simulink model "NN_PID"  (R2015a)
settings: Solver=ode45  StartTime=0.0  StopTime=40  FixedStep=0.001  RelTol=1e-3
libraries: neural x141, simulink x18, commnoisgen2 x5
(part 4 of 5)

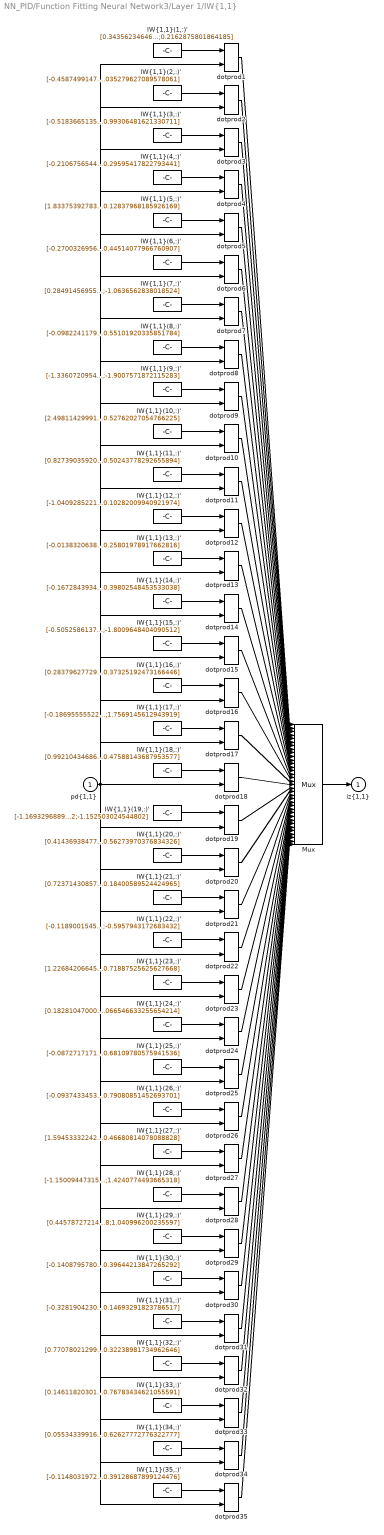
== system NN_PID/Function Fitting Neural Network3/Layer 1/IW{1,1} ==
  "pd{1,1}" : Inport  PortDimensions=20
      mask Display: e = 0.06;c1 = [120 230 180]/255;c2 = ([120 230 180]+0)/(256+128);c3 = ([120 230 180]+128)/(256+128);patch([0 1 1 0],[0 0 1 1],c1);patch([0 1 1 1-e 1-e 0+e],[0 0 1 1-e 0+e 0+e],c2);patch([0 0 1 1-e 0+e 0+e],[0 1 1 1-e 1-e 0+e],c3);plot([0 1 1 0 0],[0 0 1 1 0]);
  "IW{1,1}(1,:)'" : Constant  Value=[0.34356234646692452;0.21075488404779572;-0.32918291490554014;-0.32160977511543937;0.053207015633117721;0.43412666767247687;0.41202936590274203;0.39636100711472483;0.37639200502517606;-0.20160585970954958;0.2178319201514245;-0.15520948631781495;0.41615739491474962;-0.51184357545666392;0.38003175420582036;-0.50663702446248604;-0.33099837520790598;0.23966865807280641;0.30544580093767087;0.2162875801864185]
      mask Display: e = 0.06;c1 = [120 150 230]/255;c2 = ([120 150 230]+0)/383;c3 = ([120 150 230]+128)/383;patch([0 1 1 0],[0 0 1 1],c1);patch([0 1 1 1-e 1-e 0+e],[0 0 1 1-e 0+e 0+e],c2);patch([0 0 1 1-e 0+e 0+e],[0 1 1 1-e 1-e 0+e],c3);plot([0 1 1 0 0],[0 0 1 1 0]);disp('Weights');
  "IW{1,1}(10,:)'" : Constant  Value=[2.4981142999171224;-0.480167607602763;-0.23996584207603056;-0.53354314175989903;0.93267988161096238;-1.7895899467096461;-0.4490755724887166;-0.72970836466593303;1.6629857299245596;-1.9396925626168768;-0.017505824223907049;-0.031299172514314889;1.1546750149237817;-1.6466507506149892;0.20695638652045692;-0.69381111882218005;1.1318302015599122;-0.29293625128375828;0.58881496104867304;0.52762027054766225]
      mask Display: e = 0.06;c1 = [120 150 230]/255;c2 = ([120 150 230]+0)/383;c3 = ([120 150 230]+128)/383;patch([0 1 1 0],[0 0 1 1],c1);patch([0 1 1 1-e 1-e 0+e],[0 0 1 1-e 0+e 0+e],c2);patch([0 0 1 1-e 0+e 0+e],[0 1 1 1-e 1-e 0+e],c3);plot([0 1 1 0 0],[0 0 1 1 0]);disp('Weights');
  "IW{1,1}(11,:)'" : Constant  Value=[0.82739035920591841;0.077847341769124334;0.16416721969600542;1.3190138770003537;0.51689708649492772;0.13414226906759166;0.67634139729661547;0.29270384872245042;0.53460787889922456;0.01047726123783488;0.95499156644453731;0.15165043809919779;-0.46476741210461053;0.65252713334295698;-0.23470786792487017;0.17785522832461254;0.15426082557036538;0.51671816474315135;0.57531946627955011;-0.50243778292655894]
      mask Display: e = 0.06;c1 = [120 150 230]/255;c2 = ([120 150 230]+0)/383;c3 = ([120 150 230]+128)/383;patch([0 1 1 0],[0 0 1 1],c1);patch([0 1 1 1-e 1-e 0+e],[0 0 1 1-e 0+e 0+e],c2);patch([0 0 1 1-e 0+e 0+e],[0 1 1 1-e 1-e 0+e],c3);plot([0 1 1 0 0],[0 0 1 1 0]);disp('Weights');
  "IW{1,1}(12,:)'" : Constant  Value=[-1.0409285221258437;1.1150835262775509;-0.13810878388359787;-0.48646754358867977;-0.93383972503414348;1.572249478067455;0.25639929226933394;-0.38439956059154529;-0.70061918501654008;1.1204888375798943;0.13613187983183514;-0.58583571435844506;-1.4949035051599902;1.1826688812367208;-0.16589964378960401;-0.27085123700682673;-1.5697903319513054;0.53372313151016015;-0.20298933792670701;-0.10282009940921974]
      mask Display: e = 0.06;c1 = [120 150 230]/255;c2 = ([120 150 230]+0)/383;c3 = ([120 150 230]+128)/383;patch([0 1 1 0],[0 0 1 1],c1);patch([0 1 1 1-e 1-e 0+e],[0 0 1 1-e 0+e 0+e],c2);patch([0 0 1 1-e 0+e 0+e],[0 1 1 1-e 1-e 0+e],c3);plot([0 1 1 0 0],[0 0 1 1 0]);disp('Weights');
  "IW{1,1}(13,:)'" : Constant  Value=[-0.013832063818641063;-0.93403249848454817;-0.18601282121761561;-0.02167639873884359;0.51876133590062801;0.62596273151480519;-0.33256901492513785;0.20690823337916611;0.56369902073090317;-0.2353309824929046;0.42254575942954581;0.056199503759795696;-0.48952800638643007;-0.33465615368609403;0.490489950428382;0.50817783817270235;-0.33952374105593836;0.60950502388303041;-0.48972816769454419;-0.25801978917662816]
      mask Display: e = 0.06;c1 = [120 150 230]/255;c2 = ([120 150 230]+0)/383;c3 = ([120 150 230]+128)/383;patch([0 1 1 0],[0 0 1 1],c1);patch([0 1 1 1-e 1-e 0+e],[0 0 1 1-e 0+e 0+e],c2);patch([0 0 1 1-e 0+e 0+e],[0 1 1 1-e 1-e 0+e],c3);plot([0 1 1 0 0],[0 0 1 1 0]);disp('Weights');
  "IW{1,1}(14,:)'" : Constant  Value=[-0.16728439348193508;0.11201921876606614;-0.84717081620446133;0.033643437188791349;0.073870720164509712;0.23557579873900267;-0.47069890579339591;-0.048283879330601416;0.62682672795060768;0.3856976010503208;-1.0937018076565657;-0.24568147821005917;0.36176114292675432;0.0030879549749601026;-0.19797420086140236;0.62609705792546555;0.47665621841435707;-0.17765647171953722;0.33716085953108443;0.39802548453533038]
      mask Display: e = 0.06;c1 = [120 150 230]/255;c2 = ([120 150 230]+0)/383;c3 = ([120 150 230]+128)/383;patch([0 1 1 0],[0 0 1 1],c1);patch([0 1 1 1-e 1-e 0+e],[0 0 1 1-e 0+e 0+e],c2);patch([0 0 1 1-e 0+e 0+e],[0 1 1 1-e 1-e 0+e],c3);plot([0 1 1 0 0],[0 0 1 1 0]);disp('Weights');
  "IW{1,1}(15,:)'" : Constant  Value=[-0.50525861373297221;-0.50234172039067404;-1.0214503230073055;-0.73512099097471728;-0.88924848549223867;0.5719133518109677;-1.0086133763648022;-0.1232185415699124;-1.2092925802018386;0.097016377172541302;-0.31259485998115577;-0.38420476108191332;-0.96541704936768968;-0.79100586037197529;-0.44049745783924749;-0.23874302342060633;-0.53384968992013559;-1.0556645069035904;-1.5346677460116795;-1.8009648404090512]
      mask Display: e = 0.06;c1 = [120 150 230]/255;c2 = ([120 150 230]+0)/383;c3 = ([120 150 230]+128)/383;patch([0 1 1 0],[0 0 1 1],c1);patch([0 1 1 1-e 1-e 0+e],[0 0 1 1-e 0+e 0+e],c2);patch([0 0 1 1-e 0+e 0+e],[0 1 1 1-e 1-e 0+e],c3);plot([0 1 1 0 0],[0 0 1 1 0]);disp('Weights');
  "IW{1,1}(16,:)'" : Constant  Value=[0.28379627729071083;0.017475468939408212;0.78742097530841404;0.3402729448293319;-0.03791020600260353;0.24793319509467407;-0.14680536026554428;-0.13246445638569912;0.87176237899940057;-0.38188832490596736;0.10689208200390865;0.3257288375296703;0.076245952530720834;-0.7072342525186468;-0.54396222693874152;-0.35344510808923141;-0.559401986937623;0.39483752858509835;0.027810353114642975;0.37325192473166446]
      mask Display: e = 0.06;c1 = [120 150 230]/255;c2 = ([120 150 230]+0)/383;c3 = ([120 150 230]+128)/383;patch([0 1 1 0],[0 0 1 1],c1);patch([0 1 1 1-e 1-e 0+e],[0 0 1 1-e 0+e 0+e],c2);patch([0 0 1 1-e 0+e 0+e],[0 1 1 1-e 1-e 0+e],c3);plot([0 1 1 0 0],[0 0 1 1 0]);disp('Weights');
  "IW{1,1}(17,:)'" : Constant  Value=[-0.18695555522388208;1.1457766997082237;1.8932469743660993;1.2091852348847023;2.1793357647278508;1.5715364071793236;0.93546861520022606;1.1462136972388943;1.5547425674166264;2.1035568853621531;0.31032076523265922;-0.64150014048513371;0.98292572222818919;3.4684809472989642;1.449667710887623;2.0822190456442886;0.52834723860767396;3.448326587365893;0.66275802173830167;1.7569145612943919]
      mask Display: e = 0.06;c1 = [120 150 230]/255;c2 = ([120 150 230]+0)/383;c3 = ([120 150 230]+128)/383;patch([0 1 1 0],[0 0 1 1],c1);patch([0 1 1 1-e 1-e 0+e],[0 0 1 1-e 0+e 0+e],c2);patch([0 0 1 1-e 0+e 0+e],[0 1 1 1-e 1-e 0+e],c3);plot([0 1 1 0 0],[0 0 1 1 0]);disp('Weights');
  "IW{1,1}(18,:)'" : Constant  Value=[0.99210434686555449;-0.19182862219447805;0.83496313248633269;0.82543212806801092;-0.48831989615704796;0.17785622865467884;-0.44052762940670648;-0.93383095450336107;-1.1799218338811521;0.14631114551825533;-0.98018487699314072;-0.73495232655399023;-1.1740161013384385;0.40195376720796966;-0.68300841779666577;-0.94937235867190894;-0.72509839269384035;-0.36381020107243528;-0.56716335450951727;-0.47588143687953577]
      mask Display: e = 0.06;c1 = [120 150 230]/255;c2 = ([120 150 230]+0)/383;c3 = ([120 150 230]+128)/383;patch([0 1 1 0],[0 0 1 1],c1);patch([0 1 1 1-e 1-e 0+e],[0 0 1 1-e 0+e 0+e],c2);patch([0 0 1 1-e 0+e 0+e],[0 1 1 1-e 1-e 0+e],c3);plot([0 1 1 0 0],[0 0 1 1 0]);disp('Weights');
  "IW{1,1}(19,:)'" : Constant  Value=[-1.1693296889016684;-0.74637919668481101;-0.080745252440748996;-0.73555456972101541;-1.3624453036065594;-0.6245328994526842;-0.27615182737914001;-0.32223288713346271;-1.1053147331161475;-1.5638418877440929;0.040201830826049452;-0.69568617475109829;-1.4771542884699433;-1.384562078451685;-0.72957057859092778;-1.1255661172123617;-2.0769672387096767;-1.5456121624405867;-1.7004814221851852;-1.152503024544802]
      mask Display: e = 0.06;c1 = [120 150 230]/255;c2 = ([120 150 230]+0)/383;c3 = ([120 150 230]+128)/383;patch([0 1 1 0],[0 0 1 1],c1);patch([0 1 1 1-e 1-e 0+e],[0 0 1 1-e 0+e 0+e],c2);patch([0 0 1 1-e 0+e 0+e],[0 1 1 1-e 1-e 0+e],c3);plot([0 1 1 0 0],[0 0 1 1 0]);disp('Weights');
  "IW{1,1}(2,:)'" : Constant  Value=[-0.45874991478413735;-0.48613190251108701;-0.58937576807537073;-0.23422038712857843;-0.38105537807544038;0.15036490759582355;-0.00046876757349376651;0.4827296218033143;0.054361047774846384;0.023237702645422229;0.31821604735154824;-0.24689697381512252;0.53417251129328136;-0.46757684959937867;0.42729361373870245;-0.57415192726693309;-0.46080164770445725;0.43650630863441764;-0.0049774707672980579;0.035279627089578061]
      mask Display: e = 0.06;c1 = [120 150 230]/255;c2 = ([120 150 230]+0)/383;c3 = ([120 150 230]+128)/383;patch([0 1 1 0],[0 0 1 1],c1);patch([0 1 1 1-e 1-e 0+e],[0 0 1 1-e 0+e 0+e],c2);patch([0 0 1 1-e 0+e 0+e],[0 1 1 1-e 1-e 0+e],c3);plot([0 1 1 0 0],[0 0 1 1 0]);disp('Weights');
  "IW{1,1}(20,:)'" : Constant  Value=[0.41436938477688684;0.19335022646292935;0.014772848406684008;-0.13512928805120403;-0.063179445899241182;-0.42957513089188293;0.19337496274880683;-0.1363777958223984;0.37708859412077506;-0.025121212643982049;-0.51392570544386584;0.22904057847712325;-0.61118914251844358;0.034674346520921023;-0.41877101993291993;0.31715794586772383;0.56103736438551832;-0.01670095701532218;-0.40421432346150343;-0.56273970376834326]
      mask Display: e = 0.06;c1 = [120 150 230]/255;c2 = ([120 150 230]+0)/383;c3 = ([120 150 230]+128)/383;patch([0 1 1 0],[0 0 1 1],c1);patch([0 1 1 1-e 1-e 0+e],[0 0 1 1-e 0+e 0+e],c2);patch([0 0 1 1-e 0+e 0+e],[0 1 1 1-e 1-e 0+e],c3);plot([0 1 1 0 0],[0 0 1 1 0]);disp('Weights');
  "IW{1,1}(21,:)'" : Constant  Value=[0.72371430857203933;-3.593614507511715;-4.5871449552524277;-4.2122412121628168;0.6399350416139965;-1.818477312716956;-1.2906611084941901;-1.2875356240111187;1.123659568248192;4.3159262343879039;4.159305627556579;4.3607458437542546;0.070723338557161675;1.883176982219871;1.3223080957068787;0.86829251394765461;0.061714721775943823;0.82510572719976227;0.024549786069301308;0.18400589524424965]
      mask Display: e = 0.06;c1 = [120 150 230]/255;c2 = ([120 150 230]+0)/383;c3 = ([120 150 230]+128)/383;patch([0 1 1 0],[0 0 1 1],c1);patch([0 1 1 1-e 1-e 0+e],[0 0 1 1-e 0+e 0+e],c2);patch([0 0 1 1-e 0+e 0+e],[0 1 1 1-e 1-e 0+e],c3);plot([0 1 1 0 0],[0 0 1 1 0]);disp('Weights');
  "IW{1,1}(22,:)'" : Constant  Value=[-0.11890015452014127;-0.687701181255719;0.94376206362901938;0.23081451882508561;0.043195706054232758;0.09612049266731798;-1.1065870947943734;-0.34467190237267864;0.37138161986991153;-0.035530615058210979;-0.12065594561795193;-0.22772992194836639;0.052864999454783623;0.24879892992991279;-0.10384812085318716;-0.87109233921532081;-0.27939576841829955;0.20517011822505235;-0.16563869623528174;-0.5957943172683432]
      mask Display: e = 0.06;c1 = [120 150 230]/255;c2 = ([120 150 230]+0)/383;c3 = ([120 150 230]+128)/383;patch([0 1 1 0],[0 0 1 1],c1);patch([0 1 1 1-e 1-e 0+e],[0 0 1 1-e 0+e 0+e],c2);patch([0 0 1 1-e 0+e 0+e],[0 1 1 1-e 1-e 0+e],c3);plot([0 1 1 0 0],[0 0 1 1 0]);disp('Weights');
  "IW{1,1}(23,:)'" : Constant  Value=[1.2268420664527899;-4.7473520608111759;-4.5111987662169808;-4.1301102543078345;0.95314682285552443;-1.5369554180305878;-1.2194928954807696;-1.48885521534928;0.69535722255434684;1.1269711738240547;0.42081703079226829;-0.11006423540082071;-0.23153805097746277;3.4870735970031581;4.5861277082200518;4.686153128178999;0.23984369369556707;1.6628058364914811;0.92075306018939429;0.71887525625627668]
      mask Display: e = 0.06;c1 = [120 150 230]/255;c2 = ([120 150 230]+0)/383;c3 = ([120 150 230]+128)/383;patch([0 1 1 0],[0 0 1 1],c1);patch([0 1 1 1-e 1-e 0+e],[0 0 1 1-e 0+e 0+e],c2);patch([0 0 1 1-e 0+e 0+e],[0 1 1 1-e 1-e 0+e],c3);plot([0 1 1 0 0],[0 0 1 1 0]);disp('Weights');
  "IW{1,1}(24,:)'" : Constant  Value=[0.1828104700025977;0.31176410854197356;0.40962405803784929;-0.35642553788699693;0.057716522600453353;-0.14874504578074377;0.21254620417334505;0.46042974283685917;0.35404341798226119;0.54172712136154977;-0.58235172545159641;0.64388708858811594;-0.085376147584756507;-0.13314351100017599;-0.82733218028564015;-0.31607893422153477;0.13665134877093729;0.50278509641500502;-0.49743935447695131;0.066546633255654214]
      mask Display: e = 0.06;c1 = [120 150 230]/255;c2 = ([120 150 230]+0)/383;c3 = ([120 150 230]+128)/383;patch([0 1 1 0],[0 0 1 1],c1);patch([0 1 1 1-e 1-e 0+e],[0 0 1 1-e 0+e 0+e],c2);patch([0 0 1 1-e 0+e 0+e],[0 1 1 1-e 1-e 0+e],c3);plot([0 1 1 0 0],[0 0 1 1 0]);disp('Weights');
  "IW{1,1}(25,:)'" : Constant  Value=[-0.087271717146533007;0.11846226575201743;-0.88849593889350431;0.01343112444477061;0.23506583523325256;-0.55234171611056559;-0.47407407395654277;-0.89033223489029933;0.32638481951364251;0.085735419140751196;0.19454675867100721;0.16352631936097936;0.24207477015981532;0.40002761318930891;-0.43910346364545572;-0.084180568243685763;0.20417455686475997;0.29556820825651187;-0.9555995930734853;-0.68109780575941536]
      mask Display: e = 0.06;c1 = [120 150 230]/255;c2 = ([120 150 230]+0)/383;c3 = ([120 150 230]+128)/383;patch([0 1 1 0],[0 0 1 1],c1);patch([0 1 1 1-e 1-e 0+e],[0 0 1 1-e 0+e 0+e],c2);patch([0 0 1 1-e 0+e 0+e],[0 1 1 1-e 1-e 0+e],c3);plot([0 1 1 0 0],[0 0 1 1 0]);disp('Weights');
  "IW{1,1}(26,:)'" : Constant  Value=[-0.09374334534187008;1.3244361403553937;-0.63214199309847263;-0.8046250420468043;-0.12004482527427369;1.4122826750950541;-0.46195733135223244;-0.33569199429964125;0.6723514281939984;0.7757678158200717;-0.12247575393999316;-0.67933129844318407;0.49379968478505742;1.1284426114223642;-0.12646136822926446;-0.96154617316407409;0.4222472421730753;1.7752297376962451;-0.2198145398921153;0.79080851452693701]
      mask Display: e = 0.06;c1 = [120 150 230]/255;c2 = ([120 150 230]+0)/383;c3 = ([120 150 230]+128)/383;patch([0 1 1 0],[0 0 1 1],c1);patch([0 1 1 1-e 1-e 0+e],[0 0 1 1-e 0+e 0+e],c2);patch([0 0 1 1-e 0+e 0+e],[0 1 1 1-e 1-e 0+e],c3);plot([0 1 1 0 0],[0 0 1 1 0]);disp('Weights');
  "IW{1,1}(27,:)'" : Constant  Value=[1.5945333224281737;0.55750703331793905;0.22834970803469309;-0.55407924594364444;1.0159402558435906;0.13475888457100102;-0.94932585473437592;-0.57833908101215381;-0.21137194482521771;0.50264147781836055;-0.71057721429377341;-0.53496766081529434;0.92991557220437915;0.035881786802091149;-0.12810043583382549;0.47563250604500451;0.70661794378473586;0.15093136252852452;-0.26867178952295967;0.46680814078088828]
      mask Display: e = 0.06;c1 = [120 150 230]/255;c2 = ([120 150 230]+0)/383;c3 = ([120 150 230]+128)/383;patch([0 1 1 0],[0 0 1 1],c1);patch([0 1 1 1-e 1-e 0+e],[0 0 1 1-e 0+e 0+e],c2);patch([0 0 1 1-e 0+e 0+e],[0 1 1 1-e 1-e 0+e],c3);plot([0 1 1 0 0],[0 0 1 1 0]);disp('Weights');
  "IW{1,1}(28,:)'" : Constant  Value=[-1.1500944731533365;-0.43882767108252868;-0.51887067559486078;-0.21705590803186423;0.64998926612131047;0.074724502831834599;0.51817566210952459;0.15966122964102833;-0.5305213838452506;-0.64232198762760617;0.019688137381493213;0.7101963909482143;0.50278728648409843;-0.50395246145283856;-0.0384367465017523;0.7006560242347899;0.74282118842488443;-0.3092943056200102;1.132192267381624;1.4240774493665318]
      mask Display: e = 0.06;c1 = [120 150 230]/255;c2 = ([120 150 230]+0)/383;c3 = ([120 150 230]+128)/383;patch([0 1 1 0],[0 0 1 1],c1);patch([0 1 1 1-e 1-e 0+e],[0 0 1 1-e 0+e 0+e],c2);patch([0 0 1 1-e 0+e 0+e],[0 1 1 1-e 1-e 0+e],c3);plot([0 1 1 0 0],[0 0 1 1 0]);disp('Weights');
  "IW{1,1}(29,:)'" : Constant  Value=[0.4457872721469528;0.58517860925478815;1.5198138112088939;1.3388659684533255;1.0846180372345164;1.1710924821688653;0.20580558202619828;0.68665967354208979;0.78124105378263409;1.4629040401659914;0.18650798192964127;-0.28169842008850166;2.2921228518259875;1.336080981220338;0.63273574394653065;1.520874114106693;1.7567076375137654;1.9649644914451438;1.5521312330859938;1.040996200235597]
      mask Display: e = 0.06;c1 = [120 150 230]/255;c2 = ([120 150 230]+0)/383;c3 = ([120 150 230]+128)/383;patch([0 1 1 0],[0 0 1 1],c1);patch([0 1 1 1-e 1-e 0+e],[0 0 1 1-e 0+e 0+e],c2);patch([0 0 1 1-e 0+e 0+e],[0 1 1 1-e 1-e 0+e],c3);plot([0 1 1 0 0],[0 0 1 1 0]);disp('Weights');
  "IW{1,1}(3,:)'" : Constant  Value=[-0.51836651359350794;0.16692147273010965;0.031973839099968066;-0.26285055514279515;0.28220541671325394;-0.31185493096221517;0.02025865629207203;0.32669005765432318;0.0030836598159332731;-0.30832253903406404;-0.060331423326532442;0.73993666609635833;-0.56256953169833701;-0.70698345300566645;0.12808614394253007;0.14122723182564098;-0.48637830190550663;-0.62391538238897659;0.53003124334445673;0.99306481621330711]
      mask Display: e = 0.06;c1 = [120 150 230]/255;c2 = ([120 150 230]+0)/383;c3 = ([120 150 230]+128)/383;patch([0 1 1 0],[0 0 1 1],c1);patch([0 1 1 1-e 1-e 0+e],[0 0 1 1-e 0+e 0+e],c2);patch([0 0 1 1-e 0+e 0+e],[0 1 1 1-e 1-e 0+e],c3);plot([0 1 1 0 0],[0 0 1 1 0]);disp('Weights');
  "IW{1,1}(30,:)'" : Constant  Value=[-0.14087957801899462;0.35478617648225291;0.21149403522513699;0.41056377044908776;-0.22087054921988736;0.33497419776735021;-0.47436486406119416;-0.21221549723051042;-0.13432546537312118;0.13701637376577269;0.57805578395562429;-0.45610077329690285;0.34376937107205774;0.14500638232797852;0.44278206811243981;0.48664218987103935;0.072347278241116419;-0.24825374179427259;0.35229824512171154;-0.39644213847265292]
      mask Display: e = 0.06;c1 = [120 150 230]/255;c2 = ([120 150 230]+0)/383;c3 = ([120 150 230]+128)/383;patch([0 1 1 0],[0 0 1 1],c1);patch([0 1 1 1-e 1-e 0+e],[0 0 1 1-e 0+e 0+e],c2);patch([0 0 1 1-e 0+e 0+e],[0 1 1 1-e 1-e 0+e],c3);plot([0 1 1 0 0],[0 0 1 1 0]);disp('Weights');
  "IW{1,1}(31,:)'" : Constant  Value=[-0.32819042308196561;-0.10257381139188286;-0.37073977541966974;0.22423958924412016;-0.30795253328795763;-0.2071706128605553;-0.29040709456208469;0.082390531186220389;0.024067580871069288;0.10355229251895358;-0.13442658112358469;-0.36892314629287865;0.0045907106848744519;0.14032411420945257;-0.63942121124786999;0.15469183047235713;0.22767133858986385;-0.84477672859441388;-0.52904942613742845;0.14693291823786517]
      mask Display: e = 0.06;c1 = [120 150 230]/255;c2 = ([120 150 230]+0)/383;c3 = ([120 150 230]+128)/383;patch([0 1 1 0],[0 0 1 1],c1);patch([0 1 1 1-e 1-e 0+e],[0 0 1 1-e 0+e 0+e],c2);patch([0 0 1 1-e 0+e 0+e],[0 1 1 1-e 1-e 0+e],c3);plot([0 1 1 0 0],[0 0 1 1 0]);disp('Weights');
  "IW{1,1}(32,:)'" : Constant  Value=[0.77078021299402288;0.48081029505425493;0.21396388817095;0.12098863491066988;-0.055146482277161582;-0.39346723996023797;-0.53265112102000001;0.63390013940259193;-0.070239993932744618;0.39147026707548149;-0.12335078085922772;0.030639159154381899;-0.11383942996015066;-0.11289035557254473;-0.080150625413985321;-0.05715888336882638;0.3149151289412182;0.77859308616016143;0.085079172258503657;-0.32238981734962646]
      mask Display: e = 0.06;c1 = [120 150 230]/255;c2 = ([120 150 230]+0)/383;c3 = ([120 150 230]+128)/383;patch([0 1 1 0],[0 0 1 1],c1);patch([0 1 1 1-e 1-e 0+e],[0 0 1 1-e 0+e 0+e],c2);patch([0 0 1 1-e 0+e 0+e],[0 1 1 1-e 1-e 0+e],c3);plot([0 1 1 0 0],[0 0 1 1 0]);disp('Weights');
  "IW{1,1}(33,:)'" : Constant  Value=[0.14611820301917341;0.64966054747678437;-0.42060935671336647;-0.4822177238213004;-0.3443061873458565;0.67872546150737856;-1.2961091025588496;-0.85405600467188114;0.4144326914735576;-0.49244428450591682;-0.61602028085161153;-1.404689011803915;0.036698519057189002;-0.1393109837722625;0.23336169055112679;-0.32375828832886511;-0.32272519052731796;-0.34853452171972116;-0.013253958950352413;-0.76783434621055591]
      mask Display: e = 0.06;c1 = [120 150 230]/255;c2 = ([120 150 230]+0)/383;c3 = ([120 150 230]+128)/383;patch([0 1 1 0],[0 0 1 1],c1);patch([0 1 1 1-e 1-e 0+e],[0 0 1 1-e 0+e 0+e],c2);patch([0 0 1 1-e 0+e 0+e],[0 1 1 1-e 1-e 0+e],c3);plot([0 1 1 0 0],[0 0 1 1 0]);disp('Weights');
  "IW{1,1}(34,:)'" : Constant  Value=[0.055343399162782109;0.24967641914961913;0.22849492051757608;-0.2583701706610419;0.30234756432963239;-0.48373279085941684;-0.66349211767724392;-0.11638829875459623;0.1204720283996237;0.11020238984962738;0.48558152277647532;-0.39019701281895142;0.13510202742216729;0.23181593998038813;0.34658478847348279;0.53070352063144199;-0.40685898175808061;-0.44530896115461038;0.16484066077329629;-0.62627772776322777]
      mask Display: e = 0.06;c1 = [120 150 230]/255;c2 = ([120 150 230]+0)/383;c3 = ([120 150 230]+128)/383;patch([0 1 1 0],[0 0 1 1],c1);patch([0 1 1 1-e 1-e 0+e],[0 0 1 1-e 0+e 0+e],c2);patch([0 0 1 1-e 0+e 0+e],[0 1 1 1-e 1-e 0+e],c3);plot([0 1 1 0 0],[0 0 1 1 0]);disp('Weights');
  "IW{1,1}(35,:)'" : Constant  Value=[-0.11480319726314336;-0.5806357619062531;0.07252454074519965;-0.33034408197078352;-0.3570814673011331;-0.2053356453621932;0.055913137533546028;-0.15679935021763422;0.2825223410388083;0.35167845327504432;-0.16986653971270321;0.40801261453603693;-0.49009057489775432;0.38190469377654135;0.13229706695680551;0.45226062586800231;-0.41911899832237653;-0.25532488945121812;-0.49875611392974706;0.39128687899124476]
      mask Display: e = 0.06;c1 = [120 150 230]/255;c2 = ([120 150 230]+0)/383;c3 = ([120 150 230]+128)/383;patch([0 1 1 0],[0 0 1 1],c1);patch([0 1 1 1-e 1-e 0+e],[0 0 1 1-e 0+e 0+e],c2);patch([0 0 1 1-e 0+e 0+e],[0 1 1 1-e 1-e 0+e],c3);plot([0 1 1 0 0],[0 0 1 1 0]);disp('Weights');
  "IW{1,1}(4,:)'" : Constant  Value=[-0.21067565440528216;-0.16639612349532221;-0.89778075327033391;-1.0423459958727901;0.46816024604208872;0.25186177763045692;0.31764353669434314;0.18045330488055034;-0.18495016360448455;0.50370887995817593;0.13541207456288876;0.43565655549939025;0.4562741144442693;0.30508626067806838;-0.27852367340379708;0.34096959239955738;0.28982765605866517;0.31354521358239013;-0.089953270481375594;0.29595417822793441]
      mask Display: e = 0.06;c1 = [120 150 230]/255;c2 = ([120 150 230]+0)/383;c3 = ([120 150 230]+128)/383;patch([0 1 1 0],[0 0 1 1],c1);patch([0 1 1 1-e 1-e 0+e],[0 0 1 1-e 0+e 0+e],c2);patch([0 0 1 1-e 0+e 0+e],[0 1 1 1-e 1-e 0+e],c3);plot([0 1 1 0 0],[0 0 1 1 0]);disp('Weights');
  "IW{1,1}(5,:)'" : Constant  Value=[1.8337539278333883;0.086147383885843309;-1.4678020891736319;-0.59043101188885128;1.2472072358296118;1.0962770350027051;-0.94569854358121896;-0.43674136497767185;1.1580246739525981;0.63607980396001185;0.053375860516868545;-0.2272947020572437;0.81537950142860005;-0.25297992207888093;0.599005974575059;0.88372870065644793;0.61960905262303001;0.51200625837437308;-0.36036356482443654;-0.12837968185926169]
      mask Display: e = 0.06;c1 = [120 150 230]/255;c2 = ([120 150 230]+0)/383;c3 = ([120 150 230]+128)/383;patch([0 1 1 0],[0 0 1 1],c1);patch([0 1 1 1-e 1-e 0+e],[0 0 1 1-e 0+e 0+e],c2);patch([0 0 1 1-e 0+e 0+e],[0 1 1 1-e 1-e 0+e],c3);plot([0 1 1 0 0],[0 0 1 1 0]);disp('Weights');
  "IW{1,1}(6,:)'" : Constant  Value=[-0.2700326956327091;0.065376374079230345;0.40163042370936403;-0.31633368418214952;-0.078702611133307454;-0.70981163182088503;-0.57547631295986934;0.53870301167531431;-0.39416904709654726;-0.48975619063651638;-0.3200489975544682;-0.40405051425403499;0.065371890561165019;-0.048585089224770735;-0.44184807266874776;0.10939599677128783;0.3475544283518347;0.34605141085141949;-0.12493049943154706;0.44514077966760907]
      mask Display: e = 0.06;c1 = [120 150 230]/255;c2 = ([120 150 230]+0)/383;c3 = ([120 150 230]+128)/383;patch([0 1 1 0],[0 0 1 1],c1);patch([0 1 1 1-e 1-e 0+e],[0 0 1 1-e 0+e 0+e],c2);patch([0 0 1 1-e 0+e 0+e],[0 1 1 1-e 1-e 0+e],c3);plot([0 1 1 0 0],[0 0 1 1 0]);disp('Weights');
  "IW{1,1}(7,:)'" : Constant  Value=[0.28491456955953265;-0.53413906928550248;-2.7924099060019509;-3.3017010760226753;-0.077867633526172181;2.4105110258460773;3.1006221206099021;1.9544382422409756;-0.75472282503544874;1.976797863936959;1.2504680054747814;1.5169945297131904;-0.54357085573027963;-0.29167967914516413;0.20580430745241426;0.73838500429296494;-0.46249638008093535;-1.7805581605885168;-0.9812699185095165;-1.0636562838018524]
      mask Display: e = 0.06;c1 = [120 150 230]/255;c2 = ([120 150 230]+0)/383;c3 = ([120 150 230]+128)/383;patch([0 1 1 0],[0 0 1 1],c1);patch([0 1 1 1-e 1-e 0+e],[0 0 1 1-e 0+e 0+e],c2);patch([0 0 1 1-e 0+e 0+e],[0 1 1 1-e 1-e 0+e],c3);plot([0 1 1 0 0],[0 0 1 1 0]);disp('Weights');
  "IW{1,1}(8,:)'" : Constant  Value=[-0.098224117920649112;0.34885655019608458;0.20126106099317526;-0.27366188641622591;0.090572595783577403;-0.050946910482178455;-0.40939970109922075;-0.38103425985113343;-0.026014876775519599;0.39889802349799691;0.6812734265460717;0.25877642122681904;-0.37970226241884392;-0.38079142303390862;0.063045132094188508;-0.54327942023884856;0.14072262560426591;-0.13846896052967467;0.025559311305212166;-0.55101920335851784]
      mask Display: e = 0.06;c1 = [120 150 230]/255;c2 = ([120 150 230]+0)/383;c3 = ([120 150 230]+128)/383;patch([0 1 1 0],[0 0 1 1],c1);patch([0 1 1 1-e 1-e 0+e],[0 0 1 1-e 0+e 0+e],c2);patch([0 0 1 1-e 0+e 0+e],[0 1 1 1-e 1-e 0+e],c3);plot([0 1 1 0 0],[0 0 1 1 0]);disp('Weights');
  "IW{1,1}(9,:)'" : Constant  Value=[-1.3360720954558396;0.57903719547408616;1.0247782014349585;1.9521211577164612;-0.6188923619610549;0.12396337756632403;0.26110306732043492;-0.32160643562795588;0.54010202123575302;2.6994174378034139;3.4334678390501945;3.4933207906312753;-0.21466106315521852;-2.5966945244188455;-4.364250297590158;-4.1978017602423376;-0.88500622938410922;-0.75263665515143363;-1.9099235353683606;-1.9007571872115283]
      mask Display: e = 0.06;c1 = [120 150 230]/255;c2 = ([120 150 230]+0)/383;c3 = ([120 150 230]+128)/383;patch([0 1 1 0],[0 0 1 1],c1);patch([0 1 1 1-e 1-e 0+e],[0 0 1 1-e 0+e 0+e],c2);patch([0 0 1 1-e 0+e 0+e],[0 1 1 1-e 1-e 0+e],c3);plot([0 1 1 0 0],[0 0 1 1 0]);disp('Weights');
  Mux : Mux  Inputs=35
      mask Display: e = 0.06;c1 = [120 150 230]/255;c2 = ([120 150 230]+0)/383;c3 = ([120 150 230]+128)/383;patch([0 1 1 0],[0 0 1 1],c1);patch([0 1 1 1-e 1-e 0+e],[0 0 1 1-e 0+e 0+e],c2);patch([0 0 1 1-e 0+e 0+e],[0 1 1 1-e 1-e 0+e],c3);plot([0 1 1 0 0],[0 0 1 1 0]);disp('Mux');
  dotprod{1..35} (35 alike) : neural/Weight Functions/dotprod
  "iz{1,1}" : Outport
      mask Display: e = 0.06;c1 = [120 230 180]/255;c2 = ([120 230 180]+0)/(256+128);c3 = ([120 230 180]+128)/(256+128);patch([0 1 1 0],[0 0 1 1],c1);patch([0 1 1 1-e 1-e 0+e],[0 0 1 1-e 0+e 0+e],c2);patch([0 0 1 1-e 0+e 0+e],[0 1 1 1-e 1-e 0+e],c3);plot([0 1 1 0 0],[0 0 1 1 0]);
  wires:
  "IW{1,1}(1,:)'"/1 -> dotprod1/1
  "pd{1,1}"/1 -> dotprod1/2, dotprod2/2, dotprod3/2, dotprod4/2, dotprod5/2, dotprod6/2, dotprod7/2, dotprod8/2, dotprod9/2, dotprod10/2, dotprod11/2, dotprod12/2, dotprod13/2, dotprod14/2, dotprod15/2, dotprod16/2, dotprod17/2, dotprod18/2, dotprod19/2, dotprod20/2, dotprod21/2, dotprod22/2, dotprod23/2, dotprod24/2, dotprod25/2, dotprod26/2, dotprod27/2, dotprod28/2, dotprod29/2, dotprod30/2, dotprod31/2, dotprod32/2, dotprod33/2, dotprod34/2, dotprod35/2
  dotprod1/1 -> Mux/1
  "IW{1,1}(2,:)'"/1 -> dotprod2/1
  dotprod2/1 -> Mux/2
  "IW{1,1}(3,:)'"/1 -> dotprod3/1
  dotprod3/1 -> Mux/3
  "IW{1,1}(4,:)'"/1 -> dotprod4/1
  dotprod4/1 -> Mux/4
  "IW{1,1}(5,:)'"/1 -> dotprod5/1
  dotprod5/1 -> Mux/5
  "IW{1,1}(6,:)'"/1 -> dotprod6/1
  dotprod6/1 -> Mux/6
  "IW{1,1}(7,:)'"/1 -> dotprod7/1
  dotprod7/1 -> Mux/7
  "IW{1,1}(8,:)'"/1 -> dotprod8/1
  dotprod8/1 -> Mux/8
  "IW{1,1}(9,:)'"/1 -> dotprod9/1
  dotprod9/1 -> Mux/9
  "IW{1,1}(10,:)'"/1 -> dotprod10/1
  dotprod10/1 -> Mux/10
  "IW{1,1}(11,:)'"/1 -> dotprod11/1
  dotprod11/1 -> Mux/11
  "IW{1,1}(12,:)'"/1 -> dotprod12/1
  dotprod12/1 -> Mux/12
  "IW{1,1}(13,:)'"/1 -> dotprod13/1
  dotprod13/1 -> Mux/13
  "IW{1,1}(14,:)'"/1 -> dotprod14/1
  dotprod14/1 -> Mux/14
  "IW{1,1}(15,:)'"/1 -> dotprod15/1
  dotprod15/1 -> Mux/15
  "IW{1,1}(16,:)'"/1 -> dotprod16/1
  dotprod16/1 -> Mux/16
  "IW{1,1}(17,:)'"/1 -> dotprod17/1
  dotprod17/1 -> Mux/17
  "IW{1,1}(18,:)'"/1 -> dotprod18/1
  dotprod18/1 -> Mux/18
  "IW{1,1}(19,:)'"/1 -> dotprod19/1
  dotprod19/1 -> Mux/19
  "IW{1,1}(20,:)'"/1 -> dotprod20/1
  dotprod20/1 -> Mux/20
  "IW{1,1}(21,:)'"/1 -> dotprod21/1
  dotprod21/1 -> Mux/21
  "IW{1,1}(22,:)'"/1 -> dotprod22/1
  dotprod22/1 -> Mux/22
  "IW{1,1}(23,:)'"/1 -> dotprod23/1
  dotprod23/1 -> Mux/23
  "IW{1,1}(24,:)'"/1 -> dotprod24/1
  dotprod24/1 -> Mux/24
  "IW{1,1}(25,:)'"/1 -> dotprod25/1
  dotprod25/1 -> Mux/25
  "IW{1,1}(26,:)'"/1 -> dotprod26/1
  dotprod26/1 -> Mux/26
  "IW{1,1}(27,:)'"/1 -> dotprod27/1
  dotprod27/1 -> Mux/27
  "IW{1,1}(28,:)'"/1 -> dotprod28/1
  dotprod28/1 -> Mux/28
  "IW{1,1}(29,:)'"/1 -> dotprod29/1
  dotprod29/1 -> Mux/29
  "IW{1,1}(30,:)'"/1 -> dotprod30/1
  dotprod30/1 -> Mux/30
  "IW{1,1}(31,:)'"/1 -> dotprod31/1
  dotprod31/1 -> Mux/31
  "IW{1,1}(32,:)'"/1 -> dotprod32/1
  dotprod32/1 -> Mux/32
  "IW{1,1}(33,:)'"/1 -> dotprod33/1
  dotprod33/1 -> Mux/33
  "IW{1,1}(34,:)'"/1 -> dotprod34/1
  dotprod34/1 -> Mux/34
  "IW{1,1}(35,:)'"/1 -> dotprod35/1
  dotprod35/1 -> Mux/35
  Mux/1 -> "iz{1,1}"/1

== system NN_PID/Function Fitting Neural Network3/Layer 2/Delays 1 ==
  "p{2}" : Inport  PortDimensions=35
      mask Display: e = 0.06;c1 = [120 230 180]/255;c2 = ([120 230 180]+0)/(256+128);c3 = ([120 230 180]+128)/(256+128);patch([0 1 1 0],[0 0 1 1],c1);patch([0 1 1 1-e 1-e 0+e],[0 0 1 1-e 0+e 0+e],c2);patch([0 0 1 1-e 0+e 0+e],[0 1 1 1-e 1-e 0+e],c3);plot([0 1 1 0 0],[0 0 1 1 0]);
  mux : Mux  Inputs=1
      mask Display: e = 0.06;c1 = [120 150 230]/255;c2 = ([120 150 230]+0)/383;c3 = ([120 150 230]+128)/383;patch([0 1 1 0],[0 0 1 1],c1);patch([0 1 1 1-e 1-e 0+e],[0 0 1 1-e 0+e 0+e],c2);patch([0 0 1 1-e 0+e 0+e],[0 1 1 1-e 1-e 0+e],c3);plot([0 1 1 0 0],[0 0 1 1 0]);disp('Mux')
  "pd{2,1}" : Outport
      mask Display: e = 0.06;c1 = [120 230 180]/255;c2 = ([120 230 180]+0)/(256+128);c3 = ([120 230 180]+128)/(256+128);patch([0 1 1 0],[0 0 1 1],c1);patch([0 1 1 1-e 1-e 0+e],[0 0 1 1-e 0+e 0+e],c2);patch([0 0 1 1-e 0+e 0+e],[0 1 1 1-e 1-e 0+e],c3);plot([0 1 1 0 0],[0 0 1 1 0]);
  wires:
  "p{2}"/1 -> mux/1
  mux/1 -> "pd{2,1}"/1

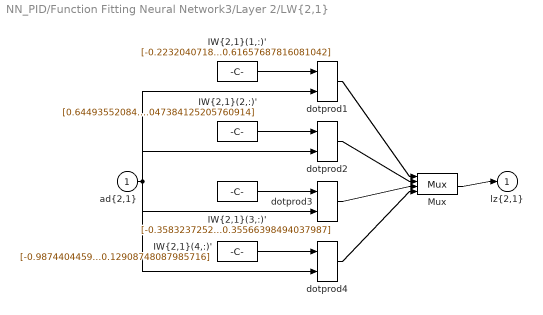
== system NN_PID/Function Fitting Neural Network3/Layer 2/LW{2,1} ==
  "ad{2,1}" : Inport  PortDimensions=35
      mask Display: e = 0.06;c1 = [120 230 180]/255;c2 = ([120 230 180]+0)/(256+128);c3 = ([120 230 180]+128)/(256+128);patch([0 1 1 0],[0 0 1 1],c1);patch([0 1 1 1-e 1-e 0+e],[0 0 1 1-e 0+e 0+e],c2);patch([0 0 1 1-e 0+e 0+e],[0 1 1 1-e 1-e 0+e],c3);plot([0 1 1 0 0],[0 0 1 1 0]);
  "IW{2,1}(1,:)'" : Constant  Value=[-0.22320407180245844;-0.24996551718941043;-0.75058630043889407;-0.99541350082695046;2.0092960308842849;0.21938585051808024;-1.3286477394165621;0.52066905631347526;-2.6453749874538364;-1.5068952121683246;1.1091723157103996;-1.486742226370775;1.0835008918139366;-0.84420917347176094;2.1628608986260245;-0.74871357851057796;1.7882528365273289;0.88867966280461652;-0.83455307312789884;0.19202960213728357;2.805461206586314;-0.88114622259938835;-3.6546278029397077;0.23171404100193158;-0.040039119738633708;-1.1356522596464838;-1.1859852067784233;1.1779431670738356;-2.3964466350033415;-0.2363938111468539;1.224788430926097;-0.86991175169181945;0.16732702009930364;0.58523106820478887;-0.61657687816081042]
      mask Display: e = 0.06;c1 = [120 150 230]/255;c2 = ([120 150 230]+0)/383;c3 = ([120 150 230]+128)/383;patch([0 1 1 0],[0 0 1 1],c1);patch([0 1 1 1-e 1-e 0+e],[0 0 1 1-e 0+e 0+e],c2);patch([0 0 1 1-e 0+e 0+e],[0 1 1 1-e 1-e 0+e],c3);plot([0 1 1 0 0],[0 0 1 1 0]);disp('weights');
  "IW{2,1}(2,:)'" : Constant  Value=[0.64493552084873962;-0.61884489171222323;0.55015093922779257;-0.26202581165388894;-2.1147098586017585;-0.58597969288750762;1.1153910114132761;0.30147370187737721;2.5055668346352382;1.902612561121898;-1.0680089807328843;2.2777129572266519;-0.32582926713124688;1.0467982450692517;-2.3837040504563629;0.023417921966313392;-2.1328269876326789;-1.1180378098887243;1.4659336536864371;0.40491683237170073;-2.6508565186835966;0.38264817662370687;3.3894714485718187;0.18896489777275771;-1.1394680224784897;0.80845828459786839;1.6907344899198267;-1.8357071801056712;3.0332274509718582;0.11529785967748847;-0.012914693838601214;0.19756175036764276;-0.65232863608775671;-0.23728537708446026;0.047384125205760914]
      mask Display: e = 0.06;c1 = [120 150 230]/255;c2 = ([120 150 230]+0)/383;c3 = ([120 150 230]+128)/383;patch([0 1 1 0],[0 0 1 1],c1);patch([0 1 1 1-e 1-e 0+e],[0 0 1 1-e 0+e 0+e],c2);patch([0 0 1 1-e 0+e 0+e],[0 1 1 1-e 1-e 0+e],c3);plot([0 1 1 0 0],[0 0 1 1 0]);disp('weights');
  "IW{2,1}(3,:)'" : Constant  Value=[-0.35832372528304629;0.47996026897504013;0.083281113530525405;0.84601075395186764;0.22635589093202027;0.56637472971771097;0.21807870392958434;0.66955531127807555;-0.28987228340658705;-1.0022761671631606;-0.20654858444558799;-0.57756184021793089;-0.45414354381583916;0.031901796274333552;-0.31025134514378194;0.28898080663741721;-0.14029890757932978;0.7879435091730107;-0.56116528209367;0.64405555253571634;-0.386423707414566;0.5298553957971488;-0.24028192384519381;0.33873582076222286;-0.35155355515153336;0.64613722383806071;-0.56994242225308178;0.67410449631776737;1.010068161955344;-0.18702856054413183;-0.49374496478657182;0.60016846853942174;-0.79764520149787932;-0.69661989873256769;0.35566398494037987]
      mask Display: e = 0.06;c1 = [120 150 230]/255;c2 = ([120 150 230]+0)/383;c3 = ([120 150 230]+128)/383;patch([0 1 1 0],[0 0 1 1],c1);patch([0 1 1 1-e 1-e 0+e],[0 0 1 1-e 0+e 0+e],c2);patch([0 0 1 1-e 0+e 0+e],[0 1 1 1-e 1-e 0+e],c3);plot([0 1 1 0 0],[0 0 1 1 0]);disp('weights');
  "IW{2,1}(4,:)'" : Constant  Value=[-0.98744044595414648;-0.072817126045275626;-0.44728693185506979;-0.82941351762360949;0.050253961395142994;-0.30184874417378271;0.78822010795994057;0.94671196787252221;-0.28618312698816234;-0.65884860645586441;0.57423572954574598;0.25579364990058406;-0.71979853245350289;-0.27245519590629563;0.58626600060053013;-0.36639869861791979;0.64783086593765149;-0.56782801447024722;-0.31415195200310531;0.39113814261095814;0.93859818122034999;-0.56187982972727413;0.31983575120289931;-0.30791106089655268;0.47077243963673315;-0.50801807264871823;-0.58750634044106709;-0.088976866025913551;-0.23117349458058073;-0.12867489254251732;0.80099695223820755;-0.30920506537983561;0.89959538463496524;0.33750431227349054;0.12908748087985716]
      mask Display: e = 0.06;c1 = [120 150 230]/255;c2 = ([120 150 230]+0)/383;c3 = ([120 150 230]+128)/383;patch([0 1 1 0],[0 0 1 1],c1);patch([0 1 1 1-e 1-e 0+e],[0 0 1 1-e 0+e 0+e],c2);patch([0 0 1 1-e 0+e 0+e],[0 1 1 1-e 1-e 0+e],c3);plot([0 1 1 0 0],[0 0 1 1 0]);disp('weights');
  Mux : Mux
      mask Display: e = 0.06;c1 = [120 150 230]/255;c2 = ([120 150 230]+0)/383;c3 = ([120 150 230]+128)/383;patch([0 1 1 0],[0 0 1 1],c1);patch([0 1 1 1-e 1-e 0+e],[0 0 1 1-e 0+e 0+e],c2);patch([0 0 1 1-e 0+e 0+e],[0 1 1 1-e 1-e 0+e],c3);plot([0 1 1 0 0],[0 0 1 1 0]);disp('Mux');
  dotprod{1..4} (4 alike) : neural/Weight Functions/dotprod
  "lz{2,1}" : Outport
      mask Display: e = 0.06;c1 = [120 230 180]/255;c2 = ([120 230 180]+0)/(256+128);c3 = ([120 230 180]+128)/(256+128);patch([0 1 1 0],[0 0 1 1],c1);patch([0 1 1 1-e 1-e 0+e],[0 0 1 1-e 0+e 0+e],c2);patch([0 0 1 1-e 0+e 0+e],[0 1 1 1-e 1-e 0+e],c3);plot([0 1 1 0 0],[0 0 1 1 0]);
  wires:
  "IW{2,1}(1,:)'"/1 -> dotprod1/1
  "ad{2,1}"/1 -> dotprod1/2, dotprod2/2, dotprod3/2, dotprod4/2
  dotprod1/1 -> Mux/1
  "IW{2,1}(2,:)'"/1 -> dotprod2/1
  dotprod2/1 -> Mux/2
  "IW{2,1}(3,:)'"/1 -> dotprod3/1
  dotprod3/1 -> Mux/3
  "IW{2,1}(4,:)'"/1 -> dotprod4/1
  dotprod4/1 -> Mux/4
  Mux/1 -> "lz{2,1}"/1

== system NN_PID/Function Fitting Neural Network4/Layer 1/Delays 1 ==
  "p{1}" : Inport  PortDimensions=32
      mask Display: e = 0.06;c1 = [120 230 180]/255;c2 = ([120 230 180]+0)/(256+128);c3 = ([120 230 180]+128)/(256+128);patch([0 1 1 0],[0 0 1 1],c1);patch([0 1 1 1-e 1-e 0+e],[0 0 1 1-e 0+e 0+e],c2);patch([0 0 1 1-e 0+e 0+e],[0 1 1 1-e 1-e 0+e],c3);plot([0 1 1 0 0],[0 0 1 1 0]);
  mux : Mux  Inputs=1
      mask Display: e = 0.06;c1 = [120 150 230]/255;c2 = ([120 150 230]+0)/383;c3 = ([120 150 230]+128)/383;patch([0 1 1 0],[0 0 1 1],c1);patch([0 1 1 1-e 1-e 0+e],[0 0 1 1-e 0+e 0+e],c2);patch([0 0 1 1-e 0+e 0+e],[0 1 1 1-e 1-e 0+e],c3);plot([0 1 1 0 0],[0 0 1 1 0]);disp('Mux')
  "pd{1,1}" : Outport
      mask Display: e = 0.06;c1 = [120 230 180]/255;c2 = ([120 230 180]+0)/(256+128);c3 = ([120 230 180]+128)/(256+128);patch([0 1 1 0],[0 0 1 1],c1);patch([0 1 1 1-e 1-e 0+e],[0 0 1 1-e 0+e 0+e],c2);patch([0 0 1 1-e 0+e 0+e],[0 1 1 1-e 1-e 0+e],c3);plot([0 1 1 0 0],[0 0 1 1 0]);
  wires:
  "p{1}"/1 -> mux/1
  mux/1 -> "pd{1,1}"/1

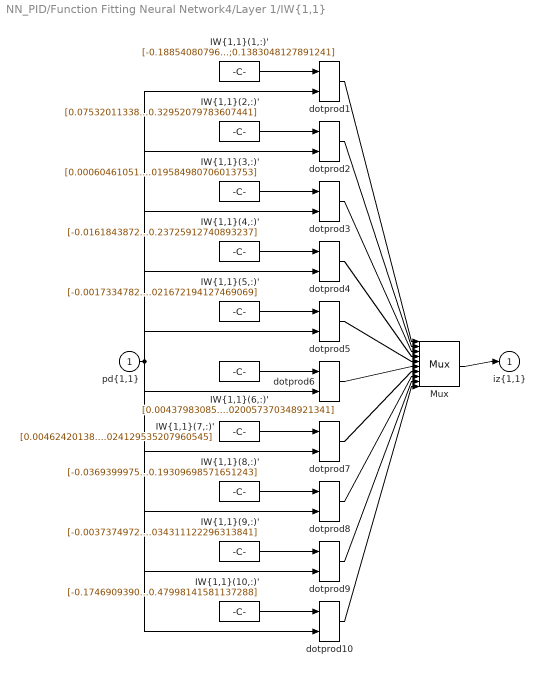
== system NN_PID/Function Fitting Neural Network4/Layer 1/IW{1,1} ==
  "pd{1,1}" : Inport  PortDimensions=32
      mask Display: e = 0.06;c1 = [120 230 180]/255;c2 = ([120 230 180]+0)/(256+128);c3 = ([120 230 180]+128)/(256+128);patch([0 1 1 0],[0 0 1 1],c1);patch([0 1 1 1-e 1-e 0+e],[0 0 1 1-e 0+e 0+e],c2);patch([0 0 1 1-e 0+e 0+e],[0 1 1 1-e 1-e 0+e],c3);plot([0 1 1 0 0],[0 0 1 1 0]);
  "IW{1,1}(1,:)'" : Constant  Value=[-0.18854080796443279;0.3543211985498011;-0.2054633842187141;0.14489074969424801;0.45698961200196125;-0.31927047730688252;0.16483072384044362;-0.2350532403353284;0.0050273968337270457;-0.43800891367533568;0.13023083021984605;0.21298593663697388;0.18724627145510633;0.061613275421696229;0.19832496040694073;0.1727490421408093;0.50982348003911226;-0.2558826838510212;-0.22207973553532434;-0.23249618566739627;-0.32551895332155778;-0.24383084677968592;-0.10150484348819827;-0.17534630171847806;0.076551938441224696;-0.24110298074320438;0.57748048715469147;0.49576896881744242;-0.18480367502770506;0.15686878561243148;0.41408719139206979;0.1383048127891241]
      mask Display: e = 0.06;c1 = [120 150 230]/255;c2 = ([120 150 230]+0)/383;c3 = ([120 150 230]+128)/383;patch([0 1 1 0],[0 0 1 1],c1);patch([0 1 1 1-e 1-e 0+e],[0 0 1 1-e 0+e 0+e],c2);patch([0 0 1 1-e 0+e 0+e],[0 1 1 1-e 1-e 0+e],c3);plot([0 1 1 0 0],[0 0 1 1 0]);disp('Weights');
  "IW{1,1}(10,:)'" : Constant  Value=[-0.17469093906920616;-0.0073833904170638844;0.16117600243557126;-0.14215716273212592;0.22377768305184995;-0.0011749117797905698;0.16331680279940436;-0.16720688379252169;-0.011861042931826242;0.12042436107628503;0.28515946599118319;-0.31805475106346515;0.27902203106631707;0.21455506950860606;0.059713674608208228;-0.09606920241882172;-0.2640160463492599;-0.32843373890608307;-0.018452481032519154;0.06635978150522856;0.27381412801962401;-0.31026338238714507;0.24619410220918161;0.97714160557609631;0.0026143992760838545;-0.035619444283671704;0.27625423678850103;0.10817995381281596;-0.26552777501494729;0.02922810210834886;0.033928664492858633;0.47998141581137288]
      mask Display: e = 0.06;c1 = [120 150 230]/255;c2 = ([120 150 230]+0)/383;c3 = ([120 150 230]+128)/383;patch([0 1 1 0],[0 0 1 1],c1);patch([0 1 1 1-e 1-e 0+e],[0 0 1 1-e 0+e 0+e],c2);patch([0 0 1 1-e 0+e 0+e],[0 1 1 1-e 1-e 0+e],c3);plot([0 1 1 0 0],[0 0 1 1 0]);disp('Weights');
  "IW{1,1}(2,:)'" : Constant  Value=[0.075320113381277573;0.12628535391121784;0.027031899773094541;-0.049594554393409922;-0.18240260269182365;-0.11764622451468373;0.18180633499732921;-0.17053906882020664;0.035368427030017663;-0.082413156034641777;0.19181763254958767;-0.15463136367876526;-0.14864102223572445;0.028703914516498535;0.051369333592613309;0.028586794281234219;0.18376886147760974;-0.055720349347263026;-0.0095101497413029642;-0.097927270864518315;-0.1577626633894024;-0.36491789289814591;-0.18904209127976618;-0.082837241602706849;-0.0090400483335159529;-0.3653189291005759;0.15556013961465637;0.31679957029340916;-0.33514903306003124;0.26972868814047318;-0.23817082094515968;-0.32952079783607441]
      mask Display: e = 0.06;c1 = [120 150 230]/255;c2 = ([120 150 230]+0)/383;c3 = ([120 150 230]+128)/383;patch([0 1 1 0],[0 0 1 1],c1);patch([0 1 1 1-e 1-e 0+e],[0 0 1 1-e 0+e 0+e],c2);patch([0 0 1 1-e 0+e 0+e],[0 1 1 1-e 1-e 0+e],c3);plot([0 1 1 0 0],[0 0 1 1 0]);disp('Weights');
  "IW{1,1}(3,:)'" : Constant  Value=[0.00060461051746328067;-0.00099288005899549861;-0.036104484799587222;0.036167887935005576;-0.00039475020884405151;0.0014240497923051953;0.1738167810237817;-0.17403079852084546;-6.8138229312844989e-05;0.00113747411987268;-0.072795977913810261;0.072318528281893474;0.00067195609382179455;0.00047624889849142641;0.3347532145680544;-0.33530357814585671;-0.0012730656840959224;-0.00034728828948296219;-0.059584009831418761;0.060341177699510119;-0.26417076003880197;-0.23304531604251066;-0.14205611299382212;0.0047763077237429593;-0.01452797443274249;-0.19191155077496283;-0.22474889060107689;-0.016408312429383825;0.023548090482708738;0.081591416680162288;0.066106894418962198;-0.019584980706013753]
      mask Display: e = 0.06;c1 = [120 150 230]/255;c2 = ([120 150 230]+0)/383;c3 = ([120 150 230]+128)/383;patch([0 1 1 0],[0 0 1 1],c1);patch([0 1 1 1-e 1-e 0+e],[0 0 1 1-e 0+e 0+e],c2);patch([0 0 1 1-e 0+e 0+e],[0 1 1 1-e 1-e 0+e],c3);plot([0 1 1 0 0],[0 0 1 1 0]);disp('Weights');
  "IW{1,1}(4,:)'" : Constant  Value=[-0.016184387289265641;-0.0021848036622333015;-0.1533570392931379;0.15477965488892587;0.025551220274523549;-0.0058321015714983028;-0.065524662778627424;0.066398135763446844;0.0037626821569962492;-0.011161389511540193;-0.0081745504596002026;0.011530220132499835;0.013361257250608941;-0.0063927035265112899;-0.21386474958544202;0.2157674295209599;-0.00011991013587902382;-0.00042541074355121559;0.23542017478281693;-0.23778080737379781;-0.09177800620126618;-0.11425425980777308;0.17606854092773366;-0.025013455103757857;-0.3540848011053504;0.21624715829363844;0.60068641040487492;0.035508068728886059;0.12363916294375898;0.0021708425905571974;0.54674570773316322;0.23725912740893237]
      mask Display: e = 0.06;c1 = [120 150 230]/255;c2 = ([120 150 230]+0)/383;c3 = ([120 150 230]+128)/383;patch([0 1 1 0],[0 0 1 1],c1);patch([0 1 1 1-e 1-e 0+e],[0 0 1 1-e 0+e 0+e],c2);patch([0 0 1 1-e 0+e 0+e],[0 1 1 1-e 1-e 0+e],c3);plot([0 1 1 0 0],[0 0 1 1 0]);disp('Weights');
  "IW{1,1}(5,:)'" : Constant  Value=[-0.0017334782435315616;-0.0019193799786332822;0.24377754316711209;-0.24357521182577851;0.0040366337497692974;0.0014903542588260959;-0.13097636004559632;0.13062028915040172;0.00070854098255702653;-0.00072600409540758909;0.30092984654703803;-0.30086043369958276;0.0030915014482164765;-0.00010616859024570757;0.17357854887805318;-0.17383755871177753;-0.0012904740582958009;-0.0010070513053959411;-0.15720257398215753;0.1574035971596463;0.36997240309339635;0.54883027738103052;-0.23344975525687695;0.0029970748186152292;-0.054579343336786032;-0.34148454247526527;-0.12698252384670186;0.032083143730410289;0.038673458682290135;0.18773755711509227;0.14932111233249629;-0.021672194127469069]
      mask Display: e = 0.06;c1 = [120 150 230]/255;c2 = ([120 150 230]+0)/383;c3 = ([120 150 230]+128)/383;patch([0 1 1 0],[0 0 1 1],c1);patch([0 1 1 1-e 1-e 0+e],[0 0 1 1-e 0+e 0+e],c2);patch([0 0 1 1-e 0+e 0+e],[0 1 1 1-e 1-e 0+e],c3);plot([0 1 1 0 0],[0 0 1 1 0]);disp('Weights');
  "IW{1,1}(6,:)'" : Constant  Value=[0.0043798308503227561;0.001826504747413908;0.23849489605322943;-0.23882358385508853;-0.0080938162343302481;0.00093704570982892867;-0.16276704058788008;0.16273048314065774;-0.0016247773224620575;0.0040357006140649705;0.23906401832106192;-0.24010957085246717;-0.0036442800724584778;0.0022091872130920362;-0.34012010073815924;0.33981923571119077;-3.0689808999510493e-05;-0.00013104612301091502;-0.26227463047612626;0.26315419028676118;-0.14893589824966133;0.25953743404526153;-0.059825615329799617;0.0095084024431574526;0.0081176798204966004;-0.022183811496709848;-0.12656098670261343;-0.13169919799943108;0.037923709308317274;-0.059360004278877838;-0.038755832018847414;-0.020057370348921341]
      mask Display: e = 0.06;c1 = [120 150 230]/255;c2 = ([120 150 230]+0)/383;c3 = ([120 150 230]+128)/383;patch([0 1 1 0],[0 0 1 1],c1);patch([0 1 1 1-e 1-e 0+e],[0 0 1 1-e 0+e 0+e],c2);patch([0 0 1 1-e 0+e 0+e],[0 1 1 1-e 1-e 0+e],c3);plot([0 1 1 0 0],[0 0 1 1 0]);disp('Weights');
  "IW{1,1}(7,:)'" : Constant  Value=[0.0046242013879265647;0.001906816610521751;-0.31343602358959216;0.31306344909573508;-0.0082589088114114438;0.00089519713222180667;-0.23054672596682355;0.23049356374850838;-0.0015250682819674044;0.0040144540884484931;-0.09851227598284551;0.097453566628185495;-0.0042477386978643792;0.0022631545417757526;0.23986604394520239;-0.2401330805386177;0.00019482229237924613;-4.4531400776769787e-05;-0.11123960672159781;0.11206756902083484;0.094547333765344507;0.018636240003128437;-0.046098775013186613;0.0092412824185008641;0.024466762376267086;-0.0013842199659149599;-0.30421934222715208;-0.1219814950701064;0.034555308762517729;-0.070932131043189545;0.084850513339899417;-0.024129535207960545]
      mask Display: e = 0.06;c1 = [120 150 230]/255;c2 = ([120 150 230]+0)/383;c3 = ([120 150 230]+128)/383;patch([0 1 1 0],[0 0 1 1],c1);patch([0 1 1 1-e 1-e 0+e],[0 0 1 1-e 0+e 0+e],c2);patch([0 0 1 1-e 0+e 0+e],[0 1 1 1-e 1-e 0+e],c3);plot([0 1 1 0 0],[0 0 1 1 0]);disp('Weights');
  "IW{1,1}(8,:)'" : Constant  Value=[-0.036939997553763752;-0.068255597533730977;-0.12062302353159937;0.13657157804116943;0.10124849637380404;0.12164372189574317;-0.22106898138258946;0.20658506966850057;-0.039733549378739144;0.06719595829857361;0.17331474637784633;-0.19641513329841259;0.078830870696617775;0.03417986429000102;-0.19010350609759905;0.13247127717812335;-0.10930877906669893;0.0047591645494354639;0.032604599071273367;0.041690546624289934;-0.29235843239379705;-0.13280606557209232;-1.0227769737900854;0.093691291439929603;-0.49265027259970195;-0.51064396850114946;0.66535956267782592;-0.31596566986123237;-0.34590019143209649;-0.40718771750049093;0.087742456585773967;-0.19309698571651243]
      mask Display: e = 0.06;c1 = [120 150 230]/255;c2 = ([120 150 230]+0)/383;c3 = ([120 150 230]+128)/383;patch([0 1 1 0],[0 0 1 1],c1);patch([0 1 1 1-e 1-e 0+e],[0 0 1 1-e 0+e 0+e],c2);patch([0 0 1 1-e 0+e 0+e],[0 1 1 1-e 1-e 0+e],c3);plot([0 1 1 0 0],[0 0 1 1 0]);disp('Weights');
  "IW{1,1}(9,:)'" : Constant  Value=[-0.0037374972197906;-0.00086534409531017695;-0.011692282741883459;0.011985458982019513;0.0060239022874117162;-0.0011165571660333236;0.013300050020196604;-0.013161459689373168;0.00091123982483841414;-0.0028932239407688859;0.36811379574159819;-0.36725751149828273;0.0033618592291107842;-0.0016718476099404907;0.15134335584388003;-0.15099201820338065;-6.7404566333305417e-06;7.03303245166639e-06;0.059379273435959466;-0.060064689230256117;0.20864668660645386;-0.24485489074612399;0.053964398280616124;-0.0070209221471450598;-0.044572003881913631;0.041787601328687557;0.33778077455712502;0.058380932291971187;-0.010279483008981065;0.025541146641053881;-0.042535759520324762;0.034311122296313841]
      mask Display: e = 0.06;c1 = [120 150 230]/255;c2 = ([120 150 230]+0)/383;c3 = ([120 150 230]+128)/383;patch([0 1 1 0],[0 0 1 1],c1);patch([0 1 1 1-e 1-e 0+e],[0 0 1 1-e 0+e 0+e],c2);patch([0 0 1 1-e 0+e 0+e],[0 1 1 1-e 1-e 0+e],c3);plot([0 1 1 0 0],[0 0 1 1 0]);disp('Weights');
  Mux : Mux  Inputs=10
      mask Display: e = 0.06;c1 = [120 150 230]/255;c2 = ([120 150 230]+0)/383;c3 = ([120 150 230]+128)/383;patch([0 1 1 0],[0 0 1 1],c1);patch([0 1 1 1-e 1-e 0+e],[0 0 1 1-e 0+e 0+e],c2);patch([0 0 1 1-e 0+e 0+e],[0 1 1 1-e 1-e 0+e],c3);plot([0 1 1 0 0],[0 0 1 1 0]);disp('Mux');
  dotprod{1..10} (10 alike) : neural/Weight Functions/dotprod
  "iz{1,1}" : Outport
      mask Display: e = 0.06;c1 = [120 230 180]/255;c2 = ([120 230 180]+0)/(256+128);c3 = ([120 230 180]+128)/(256+128);patch([0 1 1 0],[0 0 1 1],c1);patch([0 1 1 1-e 1-e 0+e],[0 0 1 1-e 0+e 0+e],c2);patch([0 0 1 1-e 0+e 0+e],[0 1 1 1-e 1-e 0+e],c3);plot([0 1 1 0 0],[0 0 1 1 0]);
  wires:
  "IW{1,1}(1,:)'"/1 -> dotprod1/1
  "pd{1,1}"/1 -> dotprod1/2, dotprod2/2, dotprod3/2, dotprod4/2, dotprod5/2, dotprod6/2, dotprod7/2, dotprod8/2, dotprod9/2, dotprod10/2
  dotprod1/1 -> Mux/1
  "IW{1,1}(2,:)'"/1 -> dotprod2/1
  dotprod2/1 -> Mux/2
  "IW{1,1}(3,:)'"/1 -> dotprod3/1
  dotprod3/1 -> Mux/3
  "IW{1,1}(4,:)'"/1 -> dotprod4/1
  dotprod4/1 -> Mux/4
  "IW{1,1}(5,:)'"/1 -> dotprod5/1
  dotprod5/1 -> Mux/5
  "IW{1,1}(6,:)'"/1 -> dotprod6/1
  dotprod6/1 -> Mux/6
  "IW{1,1}(7,:)'"/1 -> dotprod7/1
  dotprod7/1 -> Mux/7
  "IW{1,1}(8,:)'"/1 -> dotprod8/1
  dotprod8/1 -> Mux/8
  "IW{1,1}(9,:)'"/1 -> dotprod9/1
  dotprod9/1 -> Mux/9
  "IW{1,1}(10,:)'"/1 -> dotprod10/1
  dotprod10/1 -> Mux/10
  Mux/1 -> "iz{1,1}"/1

== system NN_PID/Function Fitting Neural Network4/Layer 2/Delays 1 ==
  "p{2}" : Inport  PortDimensions=10
      mask Display: e = 0.06;c1 = [120 230 180]/255;c2 = ([120 230 180]+0)/(256+128);c3 = ([120 230 180]+128)/(256+128);patch([0 1 1 0],[0 0 1 1],c1);patch([0 1 1 1-e 1-e 0+e],[0 0 1 1-e 0+e 0+e],c2);patch([0 0 1 1-e 0+e 0+e],[0 1 1 1-e 1-e 0+e],c3);plot([0 1 1 0 0],[0 0 1 1 0]);
  mux : Mux  Inputs=1
      mask Display: e = 0.06;c1 = [120 150 230]/255;c2 = ([120 150 230]+0)/383;c3 = ([120 150 230]+128)/383;patch([0 1 1 0],[0 0 1 1],c1);patch([0 1 1 1-e 1-e 0+e],[0 0 1 1-e 0+e 0+e],c2);patch([0 0 1 1-e 0+e 0+e],[0 1 1 1-e 1-e 0+e],c3);plot([0 1 1 0 0],[0 0 1 1 0]);disp('Mux')
  "pd{2,1}" : Outport
      mask Display: e = 0.06;c1 = [120 230 180]/255;c2 = ([120 230 180]+0)/(256+128);c3 = ([120 230 180]+128)/(256+128);patch([0 1 1 0],[0 0 1 1],c1);patch([0 1 1 1-e 1-e 0+e],[0 0 1 1-e 0+e 0+e],c2);patch([0 0 1 1-e 0+e 0+e],[0 1 1 1-e 1-e 0+e],c3);plot([0 1 1 0 0],[0 0 1 1 0]);
  wires:
  "p{2}"/1 -> mux/1
  mux/1 -> "pd{2,1}"/1
